simulink model "lista1_5b"  (R2020b)
settings: Solver=VariableStepAuto  StartTime=0.0  StopTime=20  RelTol=1e-3
settings Model: Creator=lucas  LastModifiedBy=lucas

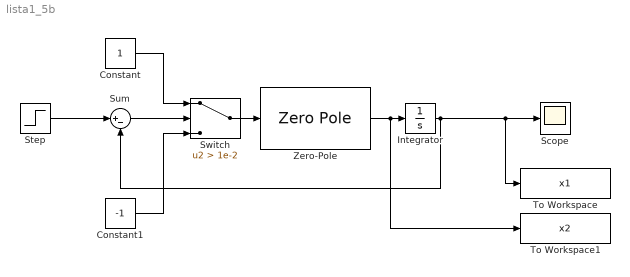
== system lista1_5b ==
  Constant : Constant
  Constant1 : Constant  Value=-1
  Integrator : Integrator
  Scope : Scope
  Step : Step  Time=0  SampleTime=0
  Sum : Sum  Inputs=|+-
  Switch : Switch  Criteria=u2 > Threshold  Threshold=1e-2
  To Workspace : ToWorkspace  VariableName=x1  SaveFormat=Timeseries  SampleTime=-1
  To Workspace1 : ToWorkspace  VariableName=x2  SaveFormat=Timeseries  SampleTime=-1
  Zero-Pole : ZeroPole  Zeros=[]  Poles=[-1 -5]  Gain=5
  wires:
  Step/1 -> Sum/1
  Sum/1 -> Switch/2
  Switch/1 -> Zero-Pole/1
  Constant/1 -> Switch/1
  Constant1/1 -> Switch/3
  Integrator/1 -> Sum/2, Scope/1, To Workspace/1
  Zero-Pole/1 -> To Workspace1/1, Integrator/1
